simulink model "buck_demo"  (R2023b)
settings: Solver=VariableStepAuto  StartTime=0.0  StopTime=Tend  RelTol=1e-3
values from neighbouring files (symbols this model uses):
  Ki = DE_out.best_sol(1,2)    [DEMO2.m]    (also in main.m)
  Kp = DE_out.best_sol(1,1)    [DEMO2.m]    (also in main.m)
  Ts = 1/Fs    (= 0.0001)    [DEMO2.m]    (also in main.m)
  Tsamp = 1/Fsamp    (= 1e-06)    [DEMO2.m]    (also in main.m)
  Ttrig = (Tstart+Tend)/2    (= 0.075)    [DEMO2.m]    (also in main.m)
  Vg = 100    [DEMO2.m]    (also in main.m)
  Vref1 = 40    [DEMO2.m]    (also in main.m)
  Vref2 = 60    [DEMO2.m]    (also in main.m)
libraries: spsSeriesRLCBranchLib x3, spsCurrentMeasurementLib x1, spsDCVoltageSourceLib x1, spsDiodeLib x1, spsMosfetLib x1, simulink x1, simulink_extras x1, spsVoltageMeasurementLib x1, sps_lib x1
settings Model: Creator=Hyeongmeen  LastModifiedBy=Hyeongmeen

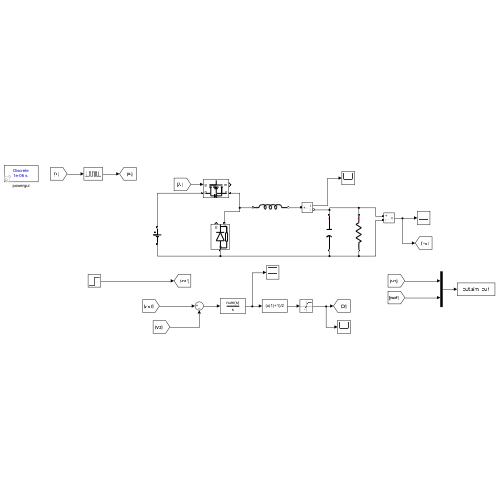
[thumbnail: Simulink's stored preview of the top-level diagram]
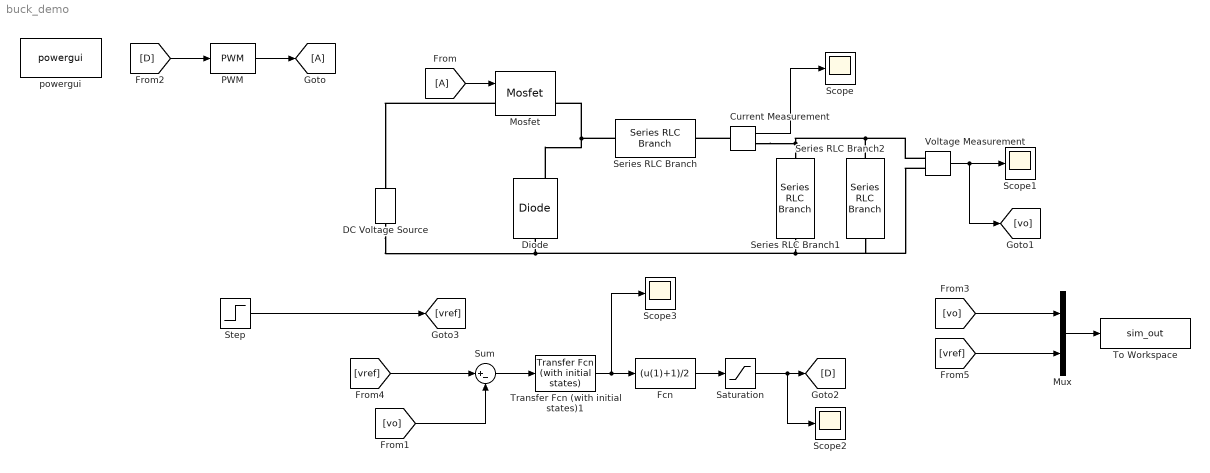
== system buck_demo ==
  Current Measurement : spsCurrentMeasurementLib/Current Measurement  PhasorSimulation=off  OutputType=Complex  PSBequivalent=0
  DC Voltage Source : spsDCVoltageSourceLib/DC Voltage Source  Amplitude=Vg  Measurements=None
  Diode : spsDiodeLib/Diode  Ron=Rdson  Lon=0  Vf=0.1  IC=0  UseSnubber=0  Rs=500  Cs=250e-9  Measurements=on
  Fcn : Fcn  Expr=(u(1)+1)/2
  From : From
  Goto : Goto
  Mosfet : spsMosfetLib/Mosfet  Ron=Rdson  Lon=0  Rd=Rdson  Vfd=0  IC=0  Rs=1e5  Cs=inf  Measurements=on
  Mux : Mux  Inputs=2
  PWM : simulink/Discontinuities/PWM  DisableCoverage=on  Period=Ts  InitialDelay=0  DisallowZeroDutyCycle=off  RunAtFixedTimeIntervals=off  SampleTime=0.1
  Saturation : Saturate  UpperLimit=1  LowerLimit=0
  Scope{,1..3} (4 alike) : Scope
  Series RLC Branch : spsSeriesRLCBranchLib/Series RLC Branch  LConnTagsString=__new0  RConnTagsString=__new0  BranchType=L  Resistance=1  Inductance=1e-3  SetiL0=off  InitialCurrent=0  Capacitance=1e-6  Setx0=off  InitialVoltage=0  Measurements=None
  Series RLC Branch1 : spsSeriesRLCBranchLib/Series RLC Branch  LConnTagsString=__new0  RConnTagsString=__new0  BranchType=C  Resistance=1  Inductance=1e-3  SetiL0=off  InitialCurrent=0  Capacitance=1e-3  Setx0=off  InitialVoltage=0  Measurements=None
  Series RLC Branch2 : spsSeriesRLCBranchLib/Series RLC Branch  LConnTagsString=__new0  RConnTagsString=__new0  BranchType=R  Resistance=1  Inductance=1e-3  SetiL0=off  InitialCurrent=0  Capacitance=1e-6  Setx0=off  InitialVoltage=0  Measurements=None
  Step : Step  Time=Ttrig  Before=Vref1  After=Vref2  SampleTime=Tsamp
  Sum : Sum  Inputs=|+-
  To Workspace : ToWorkspace  VariableName=sim_out  SaveFormat=Timeseries  SampleTime=Tsamp
  Transfer Fcn (with initial states)1 : simulink_extras/Additional Linear/Transfer Fcn (with initial states)  N=[Kp Ki]  D="[1  0]"  X0=0
  Voltage Measurement : spsVoltageMeasurementLib/Voltage Measurement  PhasorSimulation=off  OutputType=Complex  PSBequivalent=0
  powergui : sps_lib/powergui  Priority=1  SimulationMode=Discrete  SampleTime=Tsamp  frequency=60  Iterations=50  frequencyindice=0  Pbase=100e6  ErrMax=1e-4  UnitsV=kV  UnitsW=MW  buscounter=0  FunctionMessages=off  echomessages=off  EnableUseOfTLC=off  CurrentSourceSwitches=off  DisableSnubberDevices=off  DisableRonSwitches=off  DisableVfSwitches=off  DisplayEquations=off  AutomaticDiscreteSolvers=off  SolverType=Tustin/Backward Euler (TBE)  Interpol=off  ExternalGateDelay=off  methode=off  Ts=100  x0status=blocks  SPID=on  SwTol=0  HookPort=off  NonlinearTolerance=1e-4  nMaxIteration=100  ContinueOnMaxIteration=off  RestoreLinks=warning  ResistiveCurrentMeasurement=off  Frange=[0:2:500]  Ylog=off  Xlog=on  ShowGrid=off  save=off  variable=ZData  structure=0  ZoomFFT=off  StartTime=0.0  cycles=1  DisplayStyle=1  fundamental=60  FreqAxis=off  MaxFrequency=1000  frequencyindicesteady=1  RmsSteady=1  display=off
  wires:
  PWM/1 -> Goto/1
  From/1 -> Mosfet/1
  [D] -> PWM/1
  Current Measurement/1 -> Scope/1
  Voltage Measurement/1 -> [vo], Scope1/1
  [vref] -> Sum/1
  [vo] -> Sum/2
  Sum/1 -> Transfer Fcn (with initial states)1/1
  Transfer Fcn (with initial states)1/1 -> Scope3/1, Fcn/1
  Fcn/1 -> Saturation/1
  Step/1 -> [vref]
  [vo] -> Mux/1
  [vref] -> Mux/2
  Mux/1 -> To Workspace/1
  Saturation/1 -> Scope2/1, [D]
  connections:
  Mosfet/LConn1 -- DC Voltage Source/RConn1
  DC Voltage Source/LConn1 -- Voltage Measurement/LConn2 -- Series RLC Branch2/RConn1 -- Series RLC Branch1/RConn1 -- Diode/LConn1
  Diode/RConn1 -- Series RLC Branch/LConn1 -- Mosfet/RConn1
  Series RLC Branch2/LConn1 -- Voltage Measurement/LConn1 -- Current Measurement/RConn1 -- Series RLC Branch1/LConn1
  Current Measurement/LConn1 -- Series RLC Branch/RConn1
